simulink model "traffic_test"  (R2024b)
settings: Solver=VariableStepAuto  StartTime=0.0  StopTime=10.0  RelTol=1e-3
(part 2 of 2)

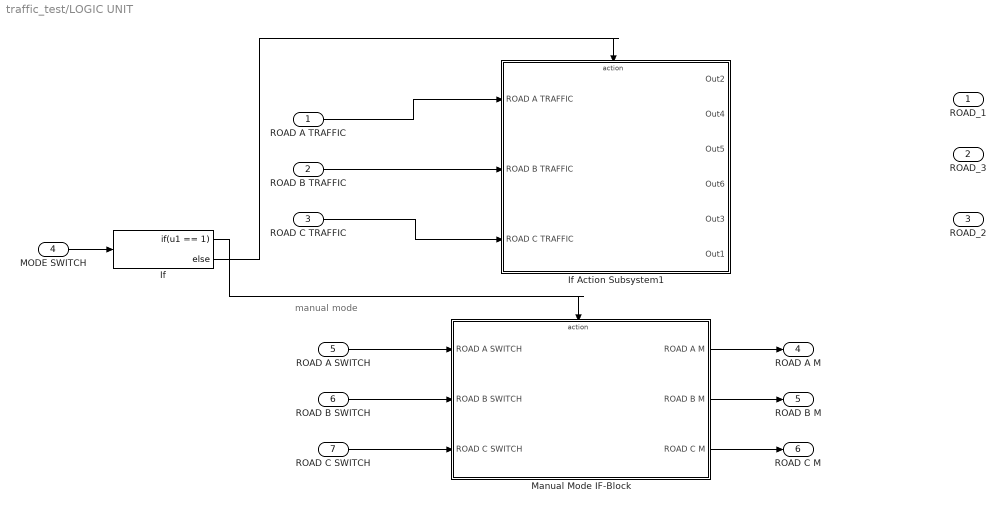
== system traffic_test/LOGIC UNIT ==
  note: manual mode
  ROAD A TRAFFIC : Inport
  ROAD B TRAFFIC : Inport  Port=2
  ROAD C TRAFFIC : Inport  Port=3
  MODE SWITCH : Inport  Port=4
  ROAD A SWITCH : Inport  Port=5
  ROAD B SWITCH : Inport  Port=6
  ROAD C SWITCH : Inport  Port=7
  If : If  IfExpression=u1 == 1
  If Action Subsystem1 : Subsystem  TreatAsAtomicUnit=on
  Manual Mode IF-Block : Subsystem  TreatAsAtomicUnit=on
  ROAD_1 : Outport
  ROAD_3 : Outport  Port=2
  ROAD_2 : Outport  Port=3
  ROAD A M : Outport  Port=4
  ROAD B M : Outport  Port=5
  ROAD C M : Outport  Port=6
  wires:
  ROAD B TRAFFIC/1 -> If Action Subsystem1/2(ROAD B TRAFFIC)
  ROAD A TRAFFIC/1 -> If Action Subsystem1/1(ROAD A TRAFFIC)
  ROAD C TRAFFIC/1 -> If Action Subsystem1/3(ROAD C TRAFFIC)
  MODE SWITCH/1 -> If/1
  If/1 -> Manual Mode IF-Block/Action
  ROAD A SWITCH/1 -> Manual Mode IF-Block/1(ROAD A SWITCH)
  ROAD B SWITCH/1 -> Manual Mode IF-Block/2(ROAD B SWITCH)
  ROAD C SWITCH/1 -> Manual Mode IF-Block/3(ROAD C SWITCH)
  If/2 -> If Action Subsystem1/Action
  Manual Mode IF-Block/1(ROAD A M) -> ROAD A M/1
  Manual Mode IF-Block/2(ROAD B M) -> ROAD B M/1
  Manual Mode IF-Block/3(ROAD C M) -> ROAD C M/1

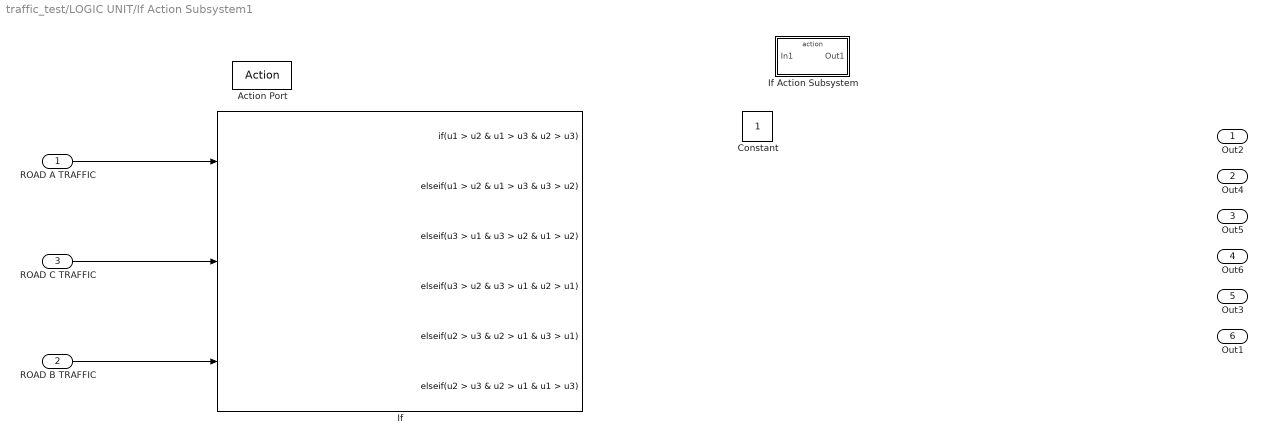
== system traffic_test/LOGIC UNIT/If Action Subsystem1 ==
  ROAD A TRAFFIC : Inport
  ROAD B TRAFFIC : Inport  Port=2
  ROAD C TRAFFIC : Inport  Port=3
  Action Port : ActionPort  ActionPortLabel=else
  Constant : Constant
  If : If  NumInputs=3  IfExpression=u1 > u2 & u1 > u3 & u2 > u3  ElseIfExpressions=u1 > u2 & u1 > u3 & u3 > u2,u3 > u1 & u3 > u2 & u1 > u2,u3 > u2 & u3 > u1 & u2 > u1,u2 > u3 & u2 > u1 & u3 > u1,u2 > u3 & u2 > u1 & u1 > u3  ShowElse=off
  If Action Subsystem : Subsystem  TreatAsAtomicUnit=on
  Out2 : Outport
  Out4 : Outport  Port=2
  Out5 : Outport  Port=3
  Out6 : Outport  Port=4
  Out3 : Outport  Port=5
  Out1 : Outport  Port=6
  wires:
  ROAD A TRAFFIC/1 -> If/1
  ROAD C TRAFFIC/1 -> If/2
  ROAD B TRAFFIC/1 -> If/3

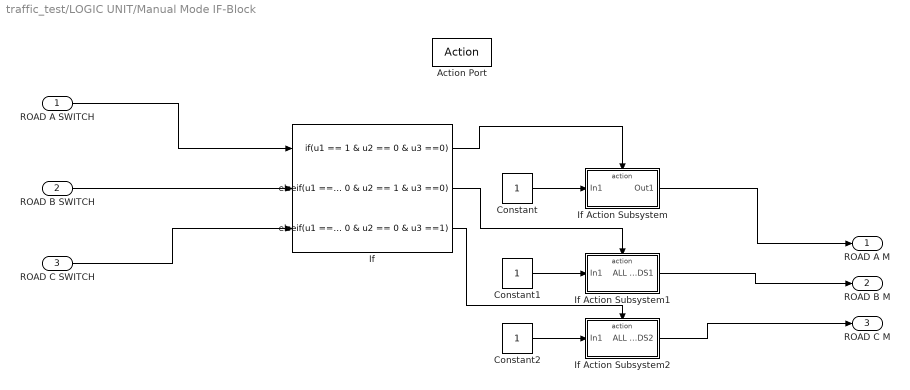
== system traffic_test/LOGIC UNIT/Manual Mode IF-Block ==
  ROAD A SWITCH : Inport
  ROAD B SWITCH : Inport  Port=2
  ROAD C SWITCH : Inport  Port=3
  Action Port : ActionPort  ActionPortLabel=if(u1 == 1)
  Constant : Constant
  Constant1 : Constant
  Constant2 : Constant
  If : If  NumInputs=3  IfExpression=u1 == 1 & u2 == 0 & u3 ==0  ElseIfExpressions=u1 == 0 & u2 == 1 & u3 ==0,u1 == 0 & u2 == 0 & u3 ==1  ShowElse=off
  If Action Subsystem : Subsystem  TreatAsAtomicUnit=on
  If Action Subsystem1 : Subsystem  TreatAsAtomicUnit=on
  If Action Subsystem2 : Subsystem  TreatAsAtomicUnit=on
  ROAD A M : Outport
  ROAD B M : Outport  Port=2
  ROAD C M : Outport  Port=3
  wires:
  ROAD A SWITCH/1 -> If/1
  ROAD B SWITCH/1 -> If/2
  ROAD C SWITCH/1 -> If/3
  If Action Subsystem/1(Out1) -> ROAD A M/1
  If/1 -> If Action Subsystem/Action
  Constant/1 -> If Action Subsystem/1(In1)
  Constant2/1 -> If Action Subsystem2/1(In1)
  If/2 -> If Action Subsystem1/Action
  If/3 -> If Action Subsystem2/Action
  Constant1/1 -> If Action Subsystem1/1(In1)
  If Action Subsystem1/1(ALL ROADS1) -> ROAD B M/1
  If Action Subsystem2/1(ALL ROADS2) -> ROAD C M/1

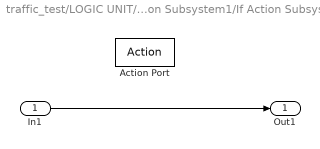
== system traffic_test/LOGIC UNIT/If Action Subsystem1/If Action Subsystem ==
  In1 : Inport
  Action Port : ActionPort
  Out1 : Outport
  wires:
  In1/1 -> Out1/1

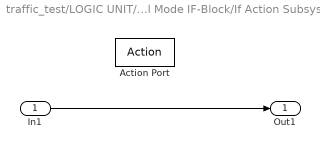
== system traffic_test/LOGIC UNIT/Manual Mode IF-Block/If Action Subsystem ==
  In1 : Inport
  Action Port : ActionPort  ActionPortLabel=if(u1 == 1 & u2 == 0 & u3 ==0)
  Out1 : Outport
  wires:
  In1/1 -> Out1/1

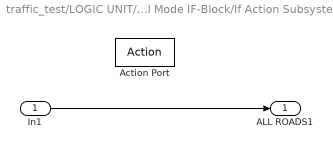
== system traffic_test/LOGIC UNIT/Manual Mode IF-Block/If Action Subsystem1 ==
  In1 : Inport
  Action Port : ActionPort  ActionPortLabel=elseif(u1 == 0 & u2 == 1 & u3 ==0)
  ALL ROADS1 : Outport
  wires:
  In1/1 -> ALL ROADS1/1

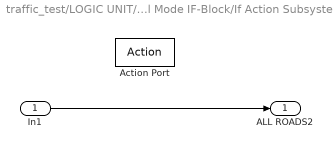
== system traffic_test/LOGIC UNIT/Manual Mode IF-Block/If Action Subsystem2 ==
  In1 : Inport
  Action Port : ActionPort  ActionPortLabel=elseif(u1 == 0 & u2 == 0 & u3 ==1)
  ALL ROADS2 : Outport
  wires:
  In1/1 -> ALL ROADS2/1
